simulink model "mass_balance_ss"  (R2025a)
settings: Solver=VariableStepAuto  StartTime=0.0  StopTime=10.0  RelTol=1e-3
libraries: nesl_utility x1
settings Model: Creator=degoede  LastModifiedBy=degoede

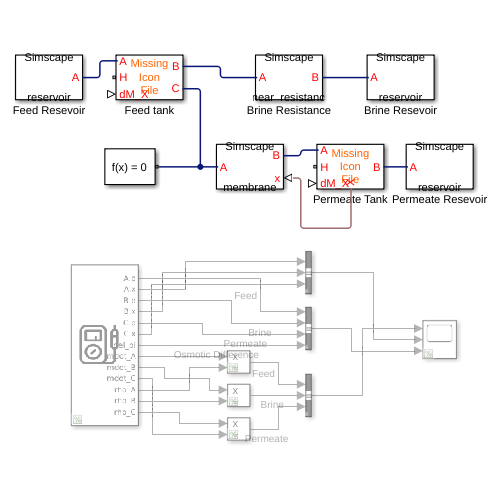
[thumbnail: Simulink's stored preview of the top-level diagram]
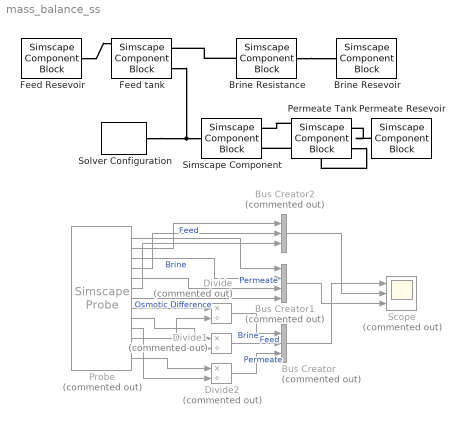
== system mass_balance_ss ==
  Brine Resevoir : SimscapeComponentBlock  SourceFile=customization.solution.elements.reservoir  ComponentPath=customization.solution.elements.reservoir  ComponentVariants="[\"customization.solution.elements.reservoir\"]"  ComponentVariantNames="[\"reservoir\"]"  ClassName=reservoir  SchemaVersion=1  pressure_spec=foundation.enum.pressure_spec.atmospheric  reservoir_pressure=0.101325 MPa  reservoir_temperature=293.15 K  reservoir_concentration=0 kg/m^3  area=0.01 m^2
      settings: CopyFcn=simscape.sscblock.internal.componentBlockCallback(gcbh,'COPY')  PreCopyFcn=simscape.sscblock.internal.componentBlockCallback(gcbh,'PRECOPY')  PreDeleteFcn=simscape.sscblock.internal.componentBlockCallback(gcbh,'PREDELETE')  InternalSimscapePortConfiguration="{\"Bottom\":[],\"Left\":[{\"id\":\"A\",\"label\":\"A\",\"type\":\"customization.solution.solution\"}],\"Right\":[],\"Top\":[]}"
      mask Type: Reservoir (SS)
  Brine Resistance : SimscapeComponentBlock  SourceFile=customization.solution.elements.linear_resistance  ComponentPath=customization.solution.elements.linear_resistance  ComponentVariants="[\"customization.solution.elements.linear_resistance\"]"  ComponentVariantNames="[\"linear_resistance\"]"  ClassName=linear_resistance  SchemaVersion=1  R=64.23e6 Pa*s/m^3  area=0.01 m^2
      settings: CopyFcn=simscape.sscblock.internal.componentBlockCallback(gcbh,'COPY')  PreCopyFcn=simscape.sscblock.internal.componentBlockCallback(gcbh,'PRECOPY')  PreDeleteFcn=simscape.sscblock.internal.componentBlockCallback(gcbh,'PREDELETE')  InternalSimscapePortConfiguration="{\"Bottom\":[],\"Left\":[{\"id\":\"A\",\"label\":\"A\",\"type\":\"customization.solution.solution\"}],\"Right\":[{\"id\":\"B\",\"label\":\"B\",\"type\":\"customization.solution.solution\"}],\"Top\":[]}"
      mask Type: Linear Resistance (SS)
  Bus Creator : BusCreator  Commented=on  Inputs=3
  Bus Creator1 : BusCreator  Commented=on  Inputs=4
  Bus Creator2 : BusCreator  Commented=on  Inputs=3
  Divide : Product  Commented=on  Inputs=*/
  Divide1 : Product  Commented=on  Inputs=*/
  Divide2 : Product  Commented=on  Inputs=*/
  Feed Resevoir : SimscapeComponentBlock  SourceFile=customization.solution.elements.reservoir  ComponentPath=customization.solution.elements.reservoir  ComponentVariants="[\"customization.solution.elements.reservoir\"]"  ComponentVariantNames="[\"reservoir\"]"  ClassName=reservoir  SchemaVersion=1  pressure_spec=foundation.enum.pressure_spec.atmospheric  reservoir_pressure=0.101325 MPa  reservoir_temperature=293.15 K  reservoir_concentration=0 kg/m^3  area=0.01 m^2
      settings: CopyFcn=simscape.sscblock.internal.componentBlockCallback(gcbh,'COPY')  PreCopyFcn=simscape.sscblock.internal.componentBlockCallback(gcbh,'PRECOPY')  PreDeleteFcn=simscape.sscblock.internal.componentBlockCallback(gcbh,'PREDELETE')  InternalSimscapePortConfiguration="{\"Bottom\":[],\"Left\":[{\"id\":\"A\",\"label\":\"A\",\"type\":\"customization.solution.solution\"}],\"Right\":[],\"Top\":[]}"
      mask Type: Reservoir (SS)
  Feed tank : SimscapeComponentBlock  SourceFile=customization.solution.elements.constant_volume_chamber  ComponentPath=customization.solution.elements.constant_volume_chamber  ComponentVariants="[\"customization.solution.elements.constant_volume_chamber\"]"  ComponentVariantNames="[\"constant_volume_chamber\"]"  ClassName=constant_volume_chamber  SchemaVersion=1  volume=0.3 m^3  num_ports=foundation.enum.num_ports.three  area_A=0.01 m^2  area_B=0.01 m^2  area_C=0.01 m^2  area_D=0.01 m^2  m_measure=false  p_measure=false  t_measure=false  x_measure=false  p_I_specify=off  p_I_priority=High  p_I=0.101325 MPa  p_I_nominal_specify=off  p_I_nominal_value=1  p_I_nominal_unit=MPa  T_I_specify=off  T_I_priority=High  T_I=293.15 K  T_I_nominal_specify=off  T_I_nominal_value=1  T_I_nominal_unit=K  u_I_specify=off  u_I_priority=None  u_I=83.906 kJ/kg  u_I_nominal_specify=off  u_I_nominal_value=1  u_I_nominal_unit=kJ/kg  rho_I_specify=off  rho_I_priority=None  rho_I=998.21 kg/m^3  rho_I_nominal_specify=off  rho_I_nominal_value=1  rho_I_nominal_unit=kg/m^3  x_I_specify=off  x_I_priority=None  x_I=0 kg/m^3  x_I_nominal_specify=off  x_I_nominal_value=1  x_I_nominal_unit=kg/m^3
      settings: CopyFcn=simscape.sscblock.internal.componentBlockCallback(gcbh,'COPY')  PreCopyFcn=simscape.sscblock.internal.componentBlockCallback(gcbh,'PRECOPY')  PreDeleteFcn=simscape.sscblock.internal.componentBlockCallback(gcbh,'PREDELETE')  InternalSimscapePortConfiguration="{\"Bottom\":[],\"Left\":[{\"id\":\"A\",\"label\":\"A\",\"type\":\"customization.solution.solution\"},{\"id\":\"H\",\"label\":\"H\",\"type\":\"foundation.thermal.thermal\"},{\"id\":\"dM_X\",\"label\":\"dM_X\",\"type\":\"input\"}],\"Right\":[{\"id\":\"B\",\"label\":\"B\",\"type\":\"customization.solution.solution\"},{\"id\":\"C\",\"label\":\"C\",\"type\":\"customization.solution.solution\"}],\"Top\":[]}"
      mask Type: Constant Volume Chamber (SS)
  Permeate Resevoir : SimscapeComponentBlock  SourceFile=customization.solution.elements.reservoir  ComponentPath=customization.solution.elements.reservoir  ComponentVariants="[\"customization.solution.elements.reservoir\"]"  ComponentVariantNames="[\"reservoir\"]"  ClassName=reservoir  SchemaVersion=1  pressure_spec=foundation.enum.pressure_spec.atmospheric  reservoir_pressure=0.101325 MPa  reservoir_temperature=293.15 K  reservoir_concentration=0 kg/m^3  area=0.01 m^2
      settings: CopyFcn=simscape.sscblock.internal.componentBlockCallback(gcbh,'COPY')  PreCopyFcn=simscape.sscblock.internal.componentBlockCallback(gcbh,'PRECOPY')  PreDeleteFcn=simscape.sscblock.internal.componentBlockCallback(gcbh,'PREDELETE')  InternalSimscapePortConfiguration="{\"Bottom\":[],\"Left\":[{\"id\":\"A\",\"label\":\"A\",\"type\":\"customization.solution.solution\"}],\"Right\":[],\"Top\":[]}"
      mask Type: Reservoir (SS)
  Permeate Tank : SimscapeComponentBlock  SourceFile=customization.solution.elements.constant_volume_chamber  ComponentPath=customization.solution.elements.constant_volume_chamber  ComponentVariants="[\"customization.solution.elements.constant_volume_chamber\"]"  ComponentVariantNames="[\"constant_volume_chamber\"]"  ClassName=constant_volume_chamber  SchemaVersion=1  volume=0.1 m^3  num_ports=foundation.enum.num_ports.two  area_A=0.01 m^2  area_B=0.01 m^2  area_C=0.01 m^2  area_D=0.01 m^2  m_measure=false  p_measure=false  t_measure=false  x_measure=true  p_I_specify=off  p_I_priority=High  p_I=0.101325 MPa  p_I_nominal_specify=off  p_I_nominal_value=1  p_I_nominal_unit=MPa  T_I_specify=off  T_I_priority=High  T_I=293.15 K  T_I_nominal_specify=off  T_I_nominal_value=1  T_I_nominal_unit=K  u_I_specify=off  u_I_priority=None  u_I=83.906 kJ/kg  u_I_nominal_specify=off  u_I_nominal_value=1  u_I_nominal_unit=kJ/kg  rho_I_specify=off  rho_I_priority=None  rho_I=998.21 kg/m^3  rho_I_nominal_specify=off  rho_I_nominal_value=1  rho_I_nominal_unit=kg/m^3  x_I_specify=off  x_I_priority=None  x_I=0 kg/m^3  x_I_nominal_specify=off  x_I_nominal_value=1  x_I_nominal_unit=kg/m^3
      settings: CopyFcn=simscape.sscblock.internal.componentBlockCallback(gcbh,'COPY')  PreCopyFcn=simscape.sscblock.internal.componentBlockCallback(gcbh,'PRECOPY')  PreDeleteFcn=simscape.sscblock.internal.componentBlockCallback(gcbh,'PREDELETE')  InternalSimscapePortConfiguration="{\"Bottom\":[{\"id\":\"X\",\"label\":\"X\",\"type\":\"output\"}],\"Left\":[{\"id\":\"A\",\"label\":\"A\",\"type\":\"customization.solution.solution\"},{\"id\":\"H\",\"label\":\"H\",\"type\":\"foundation.thermal.thermal\"},{\"id\":\"dM_X\",\"label\":\"dM_X\",\"type\":\"input\"}],\"Right\":[{\"id\":\"B\",\"label\":\"B\",\"type\":\"customization.solution.solution\"}],\"Top\":[]}"
      mask Type: Constant Volume Chamber (SS)
  Probe : SimscapeProbe  Commented=on  BoundBlock=1  Variables="{\"A.p\":{\"Probing\":\"ON\"},\"A.x\":{\"Probing\":\"ON\"},\"B.p\":{\"Probing\":\"ON\"},\"B.x\":{\"Probing\":\"ON\"},\"C.p\":{\"Probing\":\"ON\"},\"C.x\":{\"Probing\":\"ON\"},\"del_pi\":{\"Probing\":\"ON\"},\"mdot_A\":{\"Probing\":\"ON\"},\"mdot_A_x\":{\"Probing\":\"OFF\"},\"mdot_B\":{\"Probing\":\"ON\"},\"mdot_B_x\":{\"Probing\":\"OFF\"},\"mdot_C\":{\"Probing\":\"ON\"},\"mdot_C_x\":{\"Probing\":\"OFF\"},\"rho_A\":{\"Probing\":\"ON\"},\"rho_B\":{\"Probing\":\"ON\"},\"rho_C\":{\"Probing\":\"ON\"}}"
  Scope : Scope  Commented=on  NumInputPorts=3
      settings: YLabel=Flow Rate [m^3/s]
  Simscape Component : SimscapeComponentBlock  SourceFile=customization.solution.elements.membrane  ComponentPath=customization.solution.elements.membrane  ComponentVariants="[\"customization.solution.elements.membrane\"]"  ComponentVariantNames="[\"membrane\"]"  ClassName=membrane  SchemaVersion=1  A_w=2.57e-12 m^3/(N*s)  B_s=2.30e-8 m/s  A_m=35*180 m^2  area=0.01 m^2
      settings: CopyFcn=simscape.sscblock.internal.componentBlockCallback(gcbh,'COPY')  PreCopyFcn=simscape.sscblock.internal.componentBlockCallback(gcbh,'PRECOPY')  PreDeleteFcn=simscape.sscblock.internal.componentBlockCallback(gcbh,'PREDELETE')  InternalSimscapePortConfiguration="{\"Bottom\":[],\"Left\":[{\"id\":\"A\",\"label\":\"A\",\"type\":\"customization.solution.solution\"}],\"Right\":[{\"id\":\"B\",\"label\":\"B\",\"type\":\"customization.solution.solution\"},{\"id\":\"permeate_x\",\"label\":\"x\",\"type\":\"input\"}],\"Top\":[]}"
      mask Type: Membrane (SS)
  Solver Configuration : nesl_utility/Solver Configuration  PhysicalDomain=network_engine_domain  SubClassName=solver  LeftPortType=input  RightPortType=generic  Tones=[]  Harmonics=[]  SimulateNoise=off  Profile=off  UseLocalSampling=off  EnableSwitchedLinearOptims=on  FrequencyDomain=off  UseCCode=off  RelTol=0.001  AbsTol=0.001  MinStep=1e-09  ToWorkspace=off  RevertToSquareIcSolve=off  NumHomotopyIterations=100  PhasorMode=off  PhasorModeNumHarmonics=1  ConsistencySolver=NEWTON_XTOL_AFTER_FTOL  IndexReductionMethod=DerivativeReplacement  DoDC=off  ResidualTolerance=1e-09  ConsistencyTolSource=GLOBAL  ConsistencyAbsTol=0.001  ConsistencyRelTol=0.001  ConsistencyTolFactor=0.001  UseLocalSolver=off  LocalSolverChoice=NE_BACKWARD_EULER_ADVANCER  ResolveIndetEquations=on  FunctionEvalNumThread=1  LocalSolverSampleTime=0.001  DoFixedCost=off  MaxNonlinIter=3  MaxModeIter=2  ComputeImpulses=off  ImpulseIterations=2  LinearAlgebra=auto  LinearAlgebraNumThread=0  EquationFormulation=NE_TIME_EF  DelaysMemoryBudget=1024  AutomaticFiltering=on  FilteringTimeConstant=0.001  PartitionStorageMethod=AS_NEEDED  PartitionMemoryBudget=1024  PartitionMethod=ROBUST  MultibodyUseLocalSolver=off  MultibodyLocalSolverChoice=ODE1  MultibodyLocalSolverSampleTime=0.001
  wires:
  Probe/8 -> Divide/1
  Probe/9 -> Divide1/1
  Probe/13 -> Divide2/1
  Probe/10 -> Divide2/2
  Divide2/1 -> Bus Creator/3  "Permeate"
  Divide1/1 -> Bus Creator/2  "Brine"
  Divide/1 -> Bus Creator/1  "Feed"
  Probe/12 -> Divide1/2
  Probe/11 -> Divide/2
  Probe/1 -> Bus Creator1/1  "Feed"
  Probe/3 -> Bus Creator1/2  "Brine"
  Probe/5 -> Bus Creator1/3  "Permeate"
  Probe/7 -> Bus Creator1/4  "Osmotic Difference"
  Probe/2 -> Bus Creator2/1
  Probe/4 -> Bus Creator2/2
  Probe/6 -> Bus Creator2/3
  Bus Creator/1 -> Scope/1
  Bus Creator2/1 -> Scope/2
  Bus Creator1/1 -> Scope/3
  connections:
  Solver Configuration/RConn1 -- Feed tank/RConn2 -- Simscape Component/LConn1
  Brine Resistance/RConn1 -- Brine Resevoir/LConn1
  Feed Resevoir/LConn1 -- Feed tank/LConn1
  Brine Resistance/LConn1 -- Feed tank/RConn1
  Permeate Tank/LConn1 -- Simscape Component/RConn1
  Permeate Resevoir/LConn1 -- Permeate Tank/RConn1
  Permeate Tank/RConn2 -- Simscape Component/RConn2
